simulink model "sampleModel1486"  (R2023a)
settings: Solver=VariableStepAuto  StartTime=0.0  StopTime=10.0  RelTol=1e-3
libraries: hdlsllib x8, simulink x3
settings Model: Creator=user1  LastModifiedBy=user1

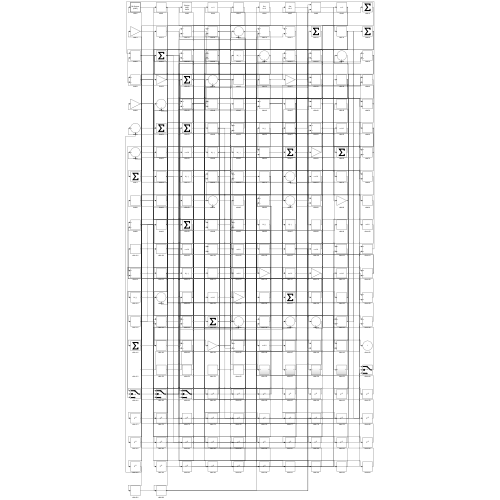
[thumbnail: Simulink's stored preview of the top-level diagram]
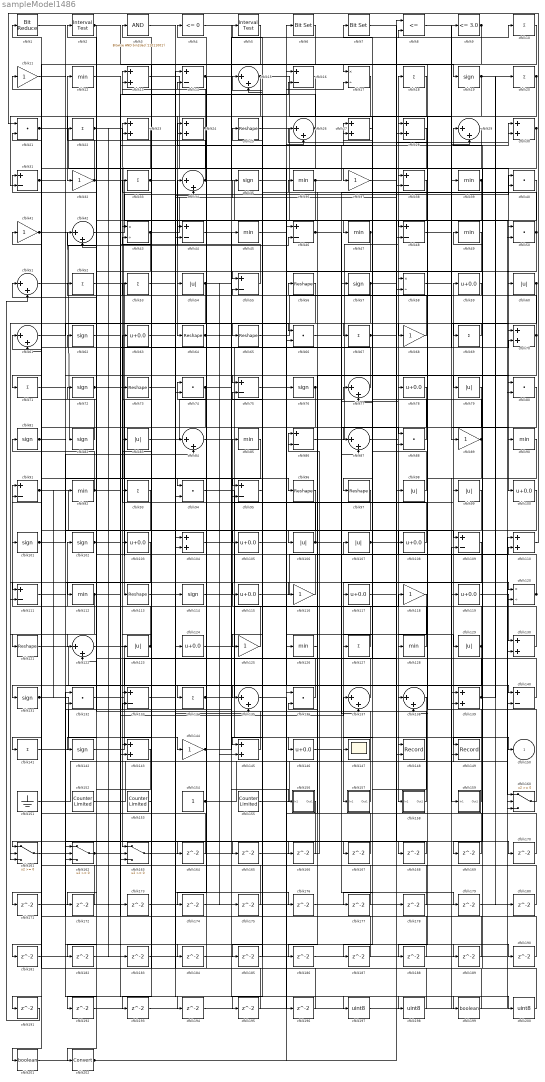
== system sampleModel1486 ==
  cfblk1 : hdlsllib/Logic and Bit Operations/Bit Reduce  mode=AND
  cfblk{10,18,20,22,33,52..53,67,69,71,93,127,134,141} (14 alike) : Sum  Inputs=+
  cfblk{59,63,78,100,103,105,108,115,117,119,124,146} (12 alike) : Bias  Bias=0.0  SaturateOnIntegerOverflow=off
  cfblk{19,35,57,62,72,76,81..82,101..102,114,131,142} (13 alike) : Signum
  cfblk{13,23..24,27..28,30,70,104,110,130,139,143,145} (13 alike) : Sum
  cfblk{54,60,79,83,98..99,106..107,123,129} (10 alike) : Abs  SaturateOnIntegerOverflow=off
  cfblk{14,16,31,38,44,46,48,55,75,86,91,95,109,111,133,140} (16 alike) : Sum  Inputs=+-
  cfblk{11,32,37,41,68,89,116,118,125,144} (10 alike) : Gain
  cfblk{12,36,39,45,47,49,85,90,92,112,126,128} (12 alike) : MinMax
  cfblk{25,56,64..65,73,96..97,113,121} (9 alike) : Reshape
  cfblk{17,43,58,120} (4 alike) : Product  Inputs=*/  RndMeth=Zero  SaturateOnIntegerOverflow=on
  cfblk{15,26,29,34,42,51,61,77,84,87,122,135,137..138} (14 alike) : Sum  Inputs=|++
  cfblk{21,40,50,66,74,80,88,94,132,136} (10 alike) : DotProduct  OutDataTypeStr=Inherit: Inherit via internal rule
  cfblk147 : Scope
  cfblk148 : Record  FileSettingsInternal="{\"entries\":[{\"content\":{\"excelSettings\":{\"content\":{},\"type\":\"Streamout.ExcelSettings\"}},\"type\":\"Streamout.FileSettingStorage\",\"uuid\":\"\"}],\"packageUris\":[\"http:\\/\\/schema.mathworks.com\\/mf0\\/streamout_blocks\\/R2020a\"],\"version\":\"1.0\"}"  Layout=[1 1]  SignalsInternal="{\"entries\":[{\"content\":{\"signals\":[{\"content\":{\"blockPath\":[],\"dimensions\":[1],\"domain\":\"\",\"lineColor\":\"#a2142f\",\"plots\":[1],\"port\":1,\"signalID\":1157,\"signalName\":\"XY Graph:1\"},\"type\":\"RecordBlkView.Signal\",\"uuid\":\"\"},{\"content\":{\"blockPath\":[],\"dimensions\":[1],\"domain\":\"\",\"lineColor\":\"#139fff\",\"plots\":[1],\"port\":2,\"signalID\":1160,\"signalName\":\"XY Graph:2\"},\"type\":\"RecordBlkView.Signal\",\"uuid\":\"\"}]},\"type\":\"RecordBlkView.InputSignals\",\"uuid\":\"\"}],\"packageUris\":[\"http:\\/\\/schema.mathworks.com\\/mf0\\/streamout_blocks\\/R2020a\"],\"version\":\"1.0\"}"  VisualizationBindings="{\"xyplotplugin\":{\"info\":[{\"series\":[{\"bindingParametersList\":[{\"parameter\":\"X-Axis\",\"signalID\":1157,\"signalName\":\"XY Graph:1\"},{\"parameter\":\"Y-Axis\",\"signalID\":1160,\"signalName\":\"XY Graph:2\"}],\"seriesID\":53532}],\"subplotID\":1}]}}"  CompatibilityTag=XY  st=-1
  cfblk149 : Record  FileSettingsInternal="{\"entries\":[{\"content\":{\"excelSettings\":{\"content\":{},\"type\":\"Streamout.ExcelSettings\"}},\"type\":\"Streamout.FileSettingStorage\",\"uuid\":\"\"}],\"packageUris\":[\"http:\\/\\/schema.mathworks.com\\/mf0\\/streamout_blocks\\/R2020a\"],\"version\":\"1.0\"}"  Layout=[1 1]  SignalsInternal="{\"entries\":[{\"content\":{\"signals\":[{\"content\":{\"blockPath\":[],\"dimensions\":[1],\"domain\":\"\",\"lineColor\":\"#a2142f\",\"plots\":[1],\"port\":1,\"signalID\":1165,\"signalName\":\"XY Graph:1\"},\"type\":\"RecordBlkView.Signal\",\"uuid\":\"\"},{\"content\":{\"blockPath\":[],\"dimensions\":[1],\"domain\":\"\",\"lineColor\":\"#139fff\",\"plots\":[1],\"port\":2,\"signalID\":1168,\"signalName\":\"XY Graph:2\"},\"type\":\"RecordBlkView.Signal\",\"uuid\":\"\"}]},\"type\":\"RecordBlkView.InputSignals\",\"uuid\":\"\"}],\"packageUris\":[\"http:\\/\\/schema.mathworks.com\\/mf0\\/streamout_blocks\\/R2020a\"],\"version\":\"1.0\"}"  VisualizationBindings="{\"xyplotplugin\":{\"info\":[{\"series\":[{\"bindingParametersList\":[{\"parameter\":\"X-Axis\",\"signalID\":1165,\"signalName\":\"XY Graph:1\"},{\"parameter\":\"Y-Axis\",\"signalID\":1168,\"signalName\":\"XY Graph:2\"}],\"seriesID\":10874}],\"subplotID\":1}]}}"  CompatibilityTag=XY  st=-1
  cfblk151 : Ground
  cfblk152 : hdlsllib/Sources/Counter Limited  uplimit=7  tsamp=-1
  cfblk153 : hdlsllib/Sources/Counter Limited  uplimit=7  tsamp=-1
  cfblk154 : Constant  SampleTime=-1
  cfblk155 : hdlsllib/Sources/Counter Limited  uplimit=7  tsamp=-1
  cfblk156 : Subsystem
      settings: LibrarySourceBlock=|
      | hdlsllib/Ports &
      | Subsystems/Subsystem
  cfblk157 : Subsystem
      settings: LibrarySourceBlock=|
      | hdlsllib/Ports &
      | Subsystems/Subsystem
  cfblk158 : Subsystem
      settings: LibrarySourceBlock=|
      | hdlsllib/Ports &
      | Subsystems/Subsystem
  cfblk159 : Subsystem
      settings: LibrarySourceBlock=|
      | hdlsllib/Ports &
      | Subsystems/Subsystem
  cfblk{160..163} (4 alike) : Switch  SaturateOnIntegerOverflow=off  InputSameDT=off
  cfblk{164..196} (33 alike) : Delay  SampleTime=1
  cfblk197 : DataTypeConversion  OutDataTypeStr=uint8  SaturateOnIntegerOverflow=off  RndMeth=Floor
  cfblk198 : DataTypeConversion  OutDataTypeStr=uint8  SaturateOnIntegerOverflow=off  RndMeth=Floor
  cfblk199 : DataTypeConversion  OutDataTypeStr=boolean  SaturateOnIntegerOverflow=off  RndMeth=Floor
  cfblk2 : hdlsllib/Logic and Bit Operations/Interval Test  IntervalClosedRight=on  uplimit=0.5  IntervalClosedLeft=on  lowlimit=-0.5  OutDataTypeStr=boolean
  cfblk200 : DataTypeConversion  OutDataTypeStr=uint8  SaturateOnIntegerOverflow=off  RndMeth=Floor
  cfblk201 : DataTypeConversion  OutDataTypeStr=boolean  SaturateOnIntegerOverflow=off  RndMeth=Floor
  cfblk202 : DataTypeConversion  SaturateOnIntegerOverflow=off  RndMeth=Floor
  cfblk3 : simulink/Logic and Bit Operations/Bitwise Operator  logicop=AND  UseBitMask=on  BitMask=bin2dec('11011001')  BitMaskRealWorld=Stored Integer
      settings: LibrarySourceBlock=|
      | hdlsllib/Logic and Bit
      | Operations/Bitwise
      | Operator
  cfblk4 : hdlsllib/Logic and Bit Operations/Compare To Zero  relop=<=  OutDataTypeStr=boolean
  cfblk5 : hdlsllib/Logic and Bit Operations/Interval Test  IntervalClosedRight=on  uplimit=0.5  IntervalClosedLeft=on  lowlimit=-0.5  OutDataTypeStr=boolean
  cfblk6 : simulink/Logic and Bit Operations/Bit Set  iBit=0
      settings: LibrarySourceBlock=|
      | hdlsllib/Logic and Bit
      | Operations/Bit Set
  cfblk7 : simulink/Logic and Bit Operations/Bit Set  iBit=0
      settings: LibrarySourceBlock=|
      | hdlsllib/Logic and Bit
      | Operations/Bit Set
  cfblk8 : RelationalOperator  Operator=<=  OutDataTypeStr=boolean  InputSameDT=off
  cfblk9 : hdlsllib/Logic and Bit Operations/Compare To Constant  relop=<=  const=3.0  OutDataTypeStr=boolean
  cfblk150 : Outport  VectorParamsAs1DForOutWhenUnconnected=off
  wires:
  cfblk28/1 -> cfblk163/1
  cfblk159/1(Out1) -> cfblk32/1
  cfblk69/1 -> cfblk65/1
  cfblk125/1 -> cfblk91/1
  cfblk52/1 -> cfblk106/1
  cfblk89/1 -> cfblk56/1, cfblk149/2
  cfblk104/1 -> cfblk136/2
  cfblk163/1 -> cfblk86/1
  cfblk22/1 -> cfblk113/1, cfblk80/1, cfblk183/1
  cfblk19/1 -> cfblk64/1, cfblk31/2, cfblk180/1, cfblk185/1
  cfblk115/1 -> cfblk18/1
  cfblk95/1 -> cfblk15/1
  cfblk64/1 -> cfblk146/1, cfblk145/2
  cfblk134/1 -> cfblk9/1, cfblk48/2
  cfblk127/1 -> cfblk85/1
  cfblk63/1 -> cfblk114/1
  cfblk25/1 -> cfblk47/1
  cfblk72/1 -> cfblk157/1(In1), cfblk173/1
  cfblk34/1 -> cfblk12/1, cfblk160/1, cfblk50/2, cfblk8/2
  cfblk14/1 -> cfblk37/1, cfblk94/1, cfblk19/1
  cfblk60/1 -> cfblk187/1, cfblk188/1
  cfblk128/1 -> cfblk41/1
  cfblk30/1 -> cfblk69/1, cfblk169/1
  cfblk86/1 -> cfblk38/1
  cfblk99/1 -> cfblk158/1(In1)
  cfblk37/1 -> cfblk30/1
  cfblk158/1(Out1) -> cfblk2/1
  cfblk29/1 -> cfblk87/1
  cfblk77/1 -> cfblk11/1
  cfblk160/1 -> cfblk26/1
  cfblk110/1 -> cfblk21/1
  cfblk151/1 -> cfblk59/1
  cfblk124/1 -> cfblk118/1
  cfblk39/1 -> cfblk67/1, cfblk97/1, cfblk143/2
  cfblk55/1 -> cfblk34/1
  cfblk122/1 -> cfblk134/1
  cfblk5/1 -> cfblk71/1
  cfblk106/1 -> cfblk63/1, cfblk78/1
  cfblk87/1 -> cfblk58/1
  cfblk32/1 -> cfblk48/1, cfblk22/1
  cfblk129/1 -> cfblk102/1, cfblk73/1, cfblk191/1
  cfblk41/1 -> cfblk82/1, cfblk80/2
  cfblk20/1 -> cfblk38/2, cfblk44/2
  cfblk130/1 -> cfblk101/1
  cfblk154/1 -> cfblk74/1, cfblk140/2
  cfblk58/1 -> cfblk89/1
  cfblk6/1 -> cfblk202/1
  cfblk68/1 -> cfblk7/1
  cfblk140/1 -> cfblk31/1
  cfblk31/1 -> cfblk79/1, cfblk115/1, cfblk184/1
  cfblk113/1 -> cfblk116/1
  cfblk94/1 -> cfblk109/1
  cfblk84/1 -> cfblk77/1
  cfblk85/1 -> cfblk121/1
  cfblk117/1 -> cfblk10/1
  cfblk120/1 -> cfblk62/1, cfblk77/2
  cfblk116/1 -> cfblk42/1
  cfblk157/1(Out1) -> cfblk83/1
  cfblk119/1 -> cfblk130/1
  cfblk27/1 -> cfblk147/1
  cfblk118/1 -> cfblk128/1
  cfblk24/1 -> cfblk74/2, cfblk13/1
  cfblk18/1 -> cfblk127/1
  cfblk10/1 -> cfblk123/1
  cfblk153/1 -> cfblk33/1
  cfblk92/1 -> cfblk81/1, cfblk27/2
  cfblk50/1 -> cfblk5/1, cfblk130/2
  cfblk13/1 -> cfblk100/1
  cfblk132/1 -> cfblk14/1
  cfblk21/1 -> cfblk126/1, cfblk163/3
  cfblk121/1 -> cfblk159/1(In1)
  cfblk141/1 -> cfblk45/1
  cfblk42/1 -> cfblk40/1
  cfblk155/1 -> cfblk87/2
  cfblk123/1 -> cfblk72/1, cfblk23/1
  cfblk91/1 -> cfblk124/1, cfblk135/1, cfblk164/1
  cfblk78/1 -> cfblk131/1
  cfblk66/1 -> cfblk88/1
  cfblk73/1 -> cfblk75/1
  cfblk38/1 -> cfblk112/1
  cfblk83/1 -> cfblk40/2
  cfblk51/1 -> cfblk46/2
  cfblk139/1 -> cfblk107/1, cfblk20/1
  cfblk62/1 -> cfblk28/1
  cfblk7/1 -> cfblk98/1
  cfblk33/1 -> cfblk84/1, cfblk135/2
  cfblk65/1 -> cfblk39/1
  cfblk114/1 -> cfblk148/1
  cfblk61/1 -> cfblk66/1
  cfblk144/1 -> cfblk99/1, cfblk168/1
  cfblk137/1 -> cfblk75/2
  cfblk9/1 -> cfblk68/1, cfblk138/2
  cfblk131/1 -> cfblk144/1, cfblk92/1
  cfblk112/1 -> cfblk161/3, cfblk16/2, cfblk199/1
  cfblk152/1 -> cfblk57/1
  cfblk101/1 -> cfblk141/1, cfblk84/2
  cfblk81/1 -> cfblk103/1, cfblk94/2
  cfblk8/1 -> cfblk70/1
  cfblk88/1 -> cfblk24/1
  cfblk54/1 -> cfblk142/1, cfblk148/2, cfblk175/1
  cfblk70/1 -> cfblk52/1, cfblk186/1
  cfblk67/1 -> cfblk27/1, cfblk170/1
  cfblk105/1 -> cfblk129/1
  cfblk40/1 -> cfblk149/1
  cfblk74/1 -> cfblk156/1(In1), cfblk143/1
  cfblk2/1 -> cfblk17/1, cfblk42/2
  cfblk109/1 -> cfblk117/1
  cfblk145/1 -> cfblk93/1
  cfblk57/1 -> cfblk28/2, cfblk111/2
  cfblk1/1 -> cfblk95/1
  cfblk71/1 -> cfblk96/1
  cfblk15/1 -> cfblk29/2, cfblk122/2
  cfblk26/1 -> cfblk43/1, cfblk13/2, cfblk111/1
  cfblk16/1 -> cfblk55/1
  cfblk142/1 -> cfblk76/1
  cfblk43/1 -> cfblk8/1, cfblk35/1, cfblk105/1, cfblk192/1
  cfblk46/1 -> cfblk139/2, cfblk50/1, cfblk137/2
  cfblk108/1 -> cfblk25/1
  cfblk126/1 -> cfblk36/1
  cfblk76/1 -> cfblk133/1, cfblk174/1
  cfblk36/1 -> cfblk125/1, cfblk30/2
  cfblk82/1 -> cfblk61/1
  cfblk59/1 -> cfblk55/2
  cfblk103/1 -> cfblk161/2
  cfblk156/1(Out1) -> cfblk162/3
  cfblk48/1 -> cfblk90/1
  cfblk162/1 -> cfblk44/1, cfblk70/2, cfblk137/1
  cfblk161/1 -> cfblk133/2
  cfblk136/1 -> cfblk51/1
  cfblk35/1 -> cfblk60/1
  cfblk90/1 -> cfblk138/1
  cfblk107/1 -> cfblk150/1, cfblk110/2
  cfblk98/1 -> cfblk53/1
  cfblk56/1 -> cfblk104/2
  cfblk17/1 -> cfblk132/2
  cfblk44/1 -> cfblk120/1
  cfblk102/1 -> cfblk189/1, cfblk198/1
  cfblk45/1 -> cfblk17/2
  cfblk47/1 -> cfblk54/1, cfblk122/1
  cfblk97/1 -> cfblk145/1
  cfblk75/1 -> cfblk140/1
  cfblk164/1 -> cfblk21/2
  cfblk49/1 -> cfblk165/1
  cfblk165/1 -> cfblk15/2
  cfblk133/1 -> cfblk166/1
  cfblk166/1 -> cfblk161/1
  cfblk12/1 -> cfblk167/1
  cfblk167/1 -> cfblk46/1
  cfblk168/1 -> cfblk162/2
  cfblk169/1 -> cfblk86/2
  cfblk170/1 -> cfblk16/1
  cfblk93/1 -> cfblk171/1
  cfblk171/1 -> cfblk136/1
  cfblk143/1 -> cfblk172/1
  cfblk172/1 -> cfblk132/1
  cfblk173/1 -> cfblk109/2
  cfblk174/1 -> cfblk160/2
  cfblk175/1 -> cfblk23/2
  cfblk53/1 -> cfblk176/1
  cfblk176/1 -> cfblk120/2
  cfblk138/1 -> cfblk177/1
  cfblk177/1 -> cfblk1/1
  cfblk178/1 -> cfblk14/2
  cfblk146/1 -> cfblk179/1
  cfblk179/1 -> cfblk29/1
  cfblk180/1 -> cfblk43/2
  cfblk79/1 -> cfblk181/1
  cfblk181/1 -> cfblk26/2
  cfblk80/1 -> cfblk182/1
  cfblk182/1 -> cfblk34/2
  cfblk183/1 -> cfblk88/2
  cfblk184/1 -> cfblk66/2
  cfblk185/1 -> cfblk95/2
  cfblk186/1 -> cfblk160/3
  cfblk187/1 -> cfblk162/1
  cfblk188/1 -> cfblk61/2
  cfblk189/1 -> cfblk24/2
  cfblk11/1 -> cfblk190/1
  cfblk190/1 -> cfblk163/2
  cfblk191/1 -> cfblk51/2
  cfblk192/1 -> cfblk58/2
  cfblk100/1 -> cfblk193/1
  cfblk193/1 -> cfblk139/1
  cfblk111/1 -> cfblk194/1
  cfblk194/1 -> cfblk110/1
  cfblk96/1 -> cfblk195/1
  cfblk195/1 -> cfblk91/2
  cfblk135/1 -> cfblk196/1
  cfblk196/1 -> cfblk104/1
  cfblk4/1 -> cfblk197/1
  cfblk197/1 -> cfblk119/1
  cfblk198/1 -> cfblk4/1
  cfblk199/1 -> cfblk3/1
  cfblk3/1 -> cfblk200/1
  cfblk200/1 -> cfblk49/1
  cfblk23/1 -> cfblk201/1
  cfblk201/1 -> cfblk6/1
  cfblk202/1 -> cfblk178/1, cfblk108/1

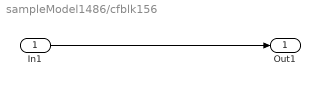
== system sampleModel1486/cfblk156 ==
  In1 : Inport
  Out1 : Outport
  wires:
  In1/1 -> Out1/1

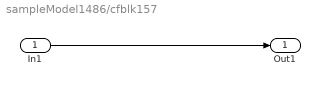
== system sampleModel1486/cfblk157 ==
  In1 : Inport
  Out1 : Outport
  wires:
  In1/1 -> Out1/1

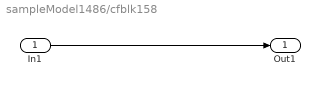
== system sampleModel1486/cfblk158 ==
  In1 : Inport
  Out1 : Outport
  wires:
  In1/1 -> Out1/1

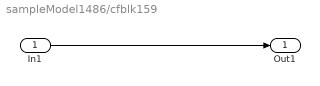
== system sampleModel1486/cfblk159 ==
  In1 : Inport
  Out1 : Outport
  wires:
  In1/1 -> Out1/1
